simulink model "orifice_model_gas"  (R2021b)
settings: Solver=VariableStepAuto  StartTime=0.0  StopTime=tsim  RelTol=1e-3
InitFcn:
  | warning 'off';
values from neighbouring files (symbols this model uses):
  do = 0.001    [script_compressor.m]    (also in script_init_pressures.m = 0.005; script_pipe_dim.m = 0.005*k/2; script_refuel.m)
  dpipe = 0.0079    [script_compressor.m]    (also in script_init_pressures.m = 0.04; script_pipe_dim.m = 0.04*k/2; script_refuel.m)
  R_h2 = 4.12    [script_H2_assumption.m]    (also in script_compressor.m; script_init_pressures.m; script_pipe_dim.m; script_refuel.m)
libraries: fl_lib x15, nesl_utility x1
(part 1 of 3)
CloseFcn:
  | try,close(h1_ssc_choked_orifice),end
  | clear h1_ssc_choked_orifice
  | 
  | clear simlog_ssc_choked_orifice tout
Description:
  | Choked Flow in Gas Orifice
  | 
  | Copyright 2016 The MathWorks, Inc.
settings Model: Creator=MathWorks  LastModifiedBy=jsagardu
settings SolverCC: AlgebraicLoopSolver=TrustRegion
settings DataIOCC: ReturnWorkspaceOutputs=off
settings DebuggingCC: SFMachineParentedDataDiag=warning  ArithmeticOperatorsInVariantConditions=warning
settings SFSimCC: SimUseLocalCustomCode=off  CustomCodeUndefinedFunction=UseInterfaceOnly
settings RTWCC: RTWUseLocalCustomCode=off
settings CodeAppCC: StateflowObjectComments=on
settings GRTTargetCC: TargetLangStandard=C89/C90 (ANSI)
settings ConfigComp: CovMetricSettings=dsw  CovSaveCumulativeToWorkspaceVar=on  CovSaveSingleToWorkspaceVar=on  CovExternalEMLEnable=off
settings SimscapeCC: SimscapeNormalizeSystem=off  SimscapeLogType=all  SimscapeLogDataHistory=10000

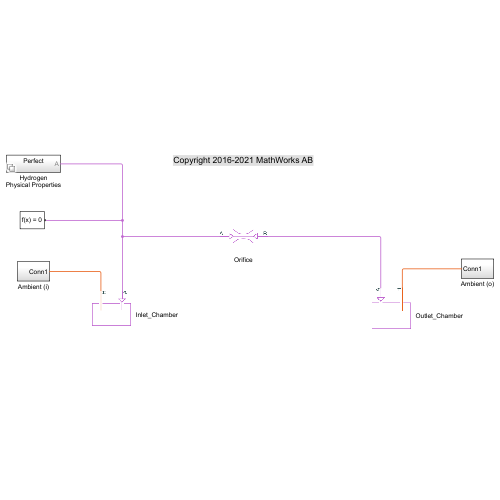
[thumbnail: Simulink's stored preview of the top-level diagram]
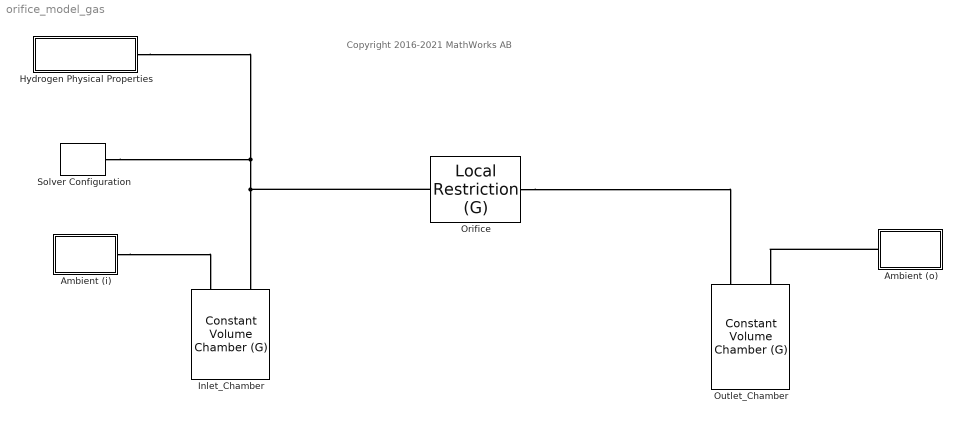
== system orifice_model_gas ==
  note: Copyright 2016-2021 MathWorks AB
  Ambient (i) : Subsystem
  Ambient (o) : Subsystem
  Hydrogen Physical Properties : Subsystem  Variant=on
  Inlet_Chamber : fl_lib/Gas/Elements/Constant Volume Chamber (G)  volume=vch_i m^3  num_ports=foundation.enum.num_ports.one  area_A=pi*dpipe^2/4 m^2  area_B=0.01 m^2  area_C=0.01 m^2  area_D=0.01 m^2  p_I_specify=on  p_I_priority=High  p_I=pi_init bar  p_I_nominal_specify=off  p_I_nominal_unit=MPa  p_I_nominal_value=1  T_I_specify=on  T_I_priority=High  T_I=Ti_init K  T_I_nominal_specify=off  T_I_nominal_unit=K  T_I_nominal_value=1  rho_chamber_specify=off  rho_chamber_priority=None  rho_chamber=1.2 kg/m^3  rho_chamber_nominal_specify=off  rho_chamber_nominal_unit=kg/m^3  rho_chamber_nominal_value=1
      settings: SourceProductBaseCode=SS  LogSimulationData=on  InternalSimscapePortConfiguration="{\"Bottom\":[],\"Left\":[{\"id\":\"A\",\"label\":\"A\",\"type\":\"foundation.gas.gas\"},{\"id\":\"H\",\"label\":\"H\",\"type\":\"foundation.thermal.thermal\"}],\"Right\":[],\"Top\":[]}"
  Orifice : fl_lib/Gas/Elements/Local Restriction (G)  restriction_type=foundation.enum.restriction_type.fixed  restriction_area=pi*do^2/4 m^2  min_area=1e-10 m^2  max_area=0.005 m^2  area=pi*dpipe^2/4 m^2  Cd=0.64  B_lam=0.999
      settings: SourceProductBaseCode=SS  InternalSimscapePortConfiguration="{\"Bottom\":[],\"Left\":[{\"id\":\"A\",\"label\":\"A\",\"type\":\"foundation.gas.gas\"}],\"Right\":[{\"id\":\"B\",\"label\":\"B\",\"type\":\"foundation.gas.gas\"}],\"Top\":[]}"
  Outlet_Chamber : fl_lib/Gas/Elements/Constant Volume Chamber (G)  volume=vch_o m^3  num_ports=foundation.enum.num_ports.one  area_A=pi*dpipe^2/4 m^2  area_B=0.01 m^2  area_C=0.01 m^2  area_D=0.01 m^2  p_I_specify=on  p_I_priority=High  p_I=po_init bar  p_I_nominal_specify=off  p_I_nominal_unit=MPa  p_I_nominal_value=1  T_I_specify=on  T_I_priority=High  T_I=To_init K  T_I_nominal_specify=off  T_I_nominal_unit=K  T_I_nominal_value=1  rho_chamber_specify=off  rho_chamber_priority=None  rho_chamber=1.2 kg/m^3  rho_chamber_nominal_specify=off  rho_chamber_nominal_unit=kg/m^3  rho_chamber_nominal_value=1
      settings: SourceProductBaseCode=SS  LogSimulationData=on  InternalSimscapePortConfiguration="{\"Bottom\":[],\"Left\":[{\"id\":\"A\",\"label\":\"A\",\"type\":\"foundation.gas.gas\"},{\"id\":\"H\",\"label\":\"H\",\"type\":\"foundation.thermal.thermal\"}],\"Right\":[],\"Top\":[]}"
  Solver Configuration : nesl_utility/Solver Configuration  PhysicalDomain=network_engine_domain  SubClassName=solver  LeftPortType=input  RightPortType=generic  Tones=[]  Harmonics=[]  SimulateNoise=off  Profile=off  UseLocalSampling=off  EnableSwitchedLinearOptims=on  FrequencyDomain=off  UseCCode=off  RelTol=0.001  AbsTol=1e-06  MinStep=1e-09  ToWorkspace=off  RevertToSquareIcSolve=off  NumHomotopyIterations=100  PhasorMode=off  PhasorModeNumHarmonics=1  DoDC=off  ResidualTolerance=1e-9  UseLocalSolver=off  LocalSolverChoice=NE_BACKWARD_EULER_ADVANCER  LocalSolverSampleTime=0.001  DoFixedCost=off  MaxNonlinIter=3  MaxModeIter=2  ComputeImpulses=off  ImpulseIterations=2  LinearAlgebra=Sparse  EquationFormulation=NE_TIME_EF  DelaysMemoryBudget=1024  AutomaticFiltering=on  FilteringTimeConstant=0.001  PartitionStorageMethod=AS_NEEDED  PartitionMemoryBudget=1024  PartitionMethod=FAST
      settings: SourceProductBaseCode=PW,SS
  connections:
  Ambient (i)/LConn1 -- Inlet_Chamber/LConn2
  Ambient (o)/LConn1 -- Outlet_Chamber/LConn2
  Hydrogen Physical Properties/RConn1 -- Inlet_Chamber/LConn1 -- Orifice/LConn1 -- Solver Configuration/RConn1
  Orifice/RConn1 -- Outlet_Chamber/LConn1

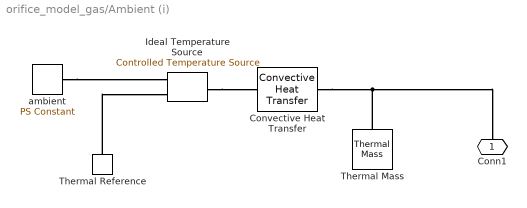
== system orifice_model_gas/Ambient (i) ==
  Convective Heat Transfer : fl_lib/Thermal/Thermal Elements/Convective Heat Transfer  area=area_ht m^2  heat_tr_coeff=alpha_ht W/(m^2 * K)  T_specify=off  T_priority=None  T=0 K  T_nominal_specify=off  T_nominal_unit=K  T_nominal_value=1  Q_specify=off  Q_priority=None  Q=0 J/s  Q_nominal_specify=off  Q_nominal_unit=W  Q_nominal_value=1
  Ideal Temperature Source : fl_lib/Thermal/Thermal Sources/Controlled Temperature Source
  Thermal Mass : fl_lib/Thermal/Thermal Elements/Thermal Mass  mass=mi kg  sp_heat=447 J/kg/K  T_specify=off  T_priority=High  T=300 K  T_nominal_specify=off  T_nominal_unit=K  T_nominal_value=1  Q_specify=off  Q_priority=None  Q=0 J/s  Q_nominal_specify=off  Q_nominal_unit=W  Q_nominal_value=1
  Thermal Reference : fl_lib/Thermal/Thermal Elements/Thermal Reference
  ambient : fl_lib/Physical Signals/Sources/PS Constant  constant=Tamb
  Conn1 : PMIOPort  Side=Left
  connections:
  Convective Heat Transfer/LConn1 -- Thermal Mass/LConn1 -- Conn1/RConn1
  Ideal Temperature Source/LConn1 -- Convective Heat Transfer/RConn1
  Thermal Reference/LConn1 -- Ideal Temperature Source/RConn2
  ambient/RConn1 -- Ideal Temperature Source/RConn1

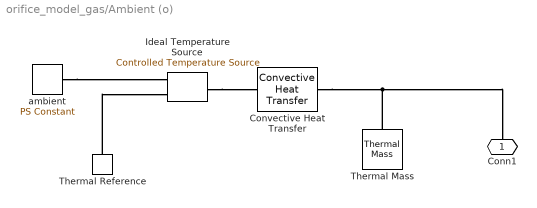
== system orifice_model_gas/Ambient (o) ==
  Convective Heat Transfer : fl_lib/Thermal/Thermal Elements/Convective Heat Transfer  area=area_ht m^2  heat_tr_coeff=alpha_ht W/(m^2 * K)  T_specify=off  T_priority=None  T=0 K  T_nominal_specify=off  T_nominal_unit=K  T_nominal_value=1  Q_specify=off  Q_priority=None  Q=0 J/s  Q_nominal_specify=off  Q_nominal_unit=W  Q_nominal_value=1
  Ideal Temperature Source : fl_lib/Thermal/Thermal Sources/Controlled Temperature Source
  Thermal Mass : fl_lib/Thermal/Thermal Elements/Thermal Mass  mass=mo kg  sp_heat=447 J/kg/K  T_specify=off  T_priority=High  T=300 K  T_nominal_specify=off  T_nominal_unit=K  T_nominal_value=1  Q_specify=off  Q_priority=None  Q=0 J/s  Q_nominal_specify=off  Q_nominal_unit=W  Q_nominal_value=1
  Thermal Reference : fl_lib/Thermal/Thermal Elements/Thermal Reference
  ambient : fl_lib/Physical Signals/Sources/PS Constant  constant=Tamb
  Conn1 : PMIOPort  Side=Left
  connections:
  Convective Heat Transfer/LConn1 -- Thermal Mass/LConn1 -- Conn1/RConn1
  Ideal Temperature Source/LConn1 -- Convective Heat Transfer/RConn1
  Thermal Reference/LConn1 -- Ideal Temperature Source/RConn2
  ambient/RConn1 -- Ideal Temperature Source/RConn1

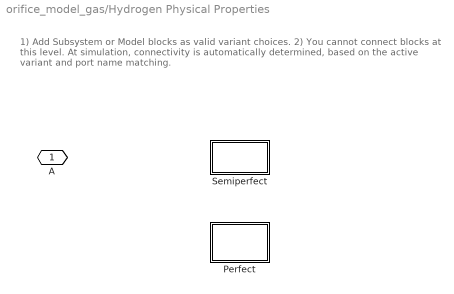
== system orifice_model_gas/Hydrogen Physical Properties ==
  note: 1) Add Subsystem or Model blocks as valid variant choices.
      | 2) You cannot connect blocks at this level. At simulation, connectivity is automatically
      | determined, based on the active variant and port name matching.
  Perfect : Subsystem  VariantControl=var_a>0
  Semiperfect : Subsystem  VariantControl=var_b>0
  A : PMIOPort  Side=Right
